simulink model "sim8"  (R2013a)
settings: Solver=ode45  StartTime=0.0  StopTime=10.0  RelTol=1e-3
values from neighbouring files (symbols this model uses):
  a1 = 4    [cwiczenie8.m]    (also in cwiczenie8transmitancja.m)
  A1 = 2    [cwiczenie8.m]    (also in cwiczenie8transmitancja.m; dawid.m)
  A2 = 4    [cwiczenie8.m]    (also in cwiczenie8transmitancja.m; dawid.m)
  a2 = 5    [cwiczenie8.m]    (also in cwiczenie8transmitancja.m)
  czas_skoku = 2    [cwiczenie8.m]    (also in cwiczenie8transmitancja.m; dawid.m)
  du = 0.1*u0max    (= 0.3)    [cwiczenie8.m]    (also in cwiczenie8transmitancja.m; dawid.m)
  h10 = u0/a1    [cwiczenie8.m]    (also in cwiczenie8transmitancja.m; dawid.m = u0*u0 / (Awy*Awy*2*g))
  h20 = u0/a2    [cwiczenie8.m]    (also in cwiczenie8transmitancja.m; dawid.m = u0*u0 / (Awe*Awe*2*g))
  u0 = tabu0(i)    [cwiczenie8.m]    (also in cwiczenie8transmitancja.m; dawid.m)
settings Model: Creator=LAB320-1552  LastModifiedBy=LAB320-1552

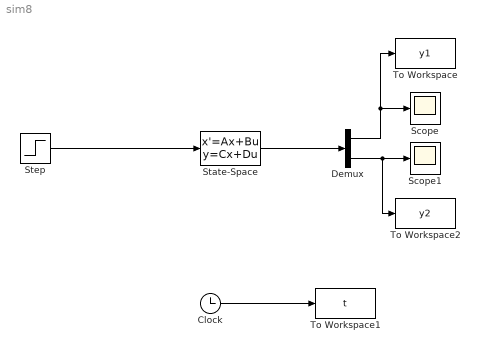
== system sim8 ==
  Clock : Clock
  Demux : Demux  Outputs=2
  Scope : Scope
  Scope1 : Scope
  State-Space : StateSpace  A=[-a1/A1, 0; a1/A2, -a2/A2]  B=[1/A1; 0]  C=[1, 0; 0, 1]  D=[0; 0]  X0=[h10; h20]
  Step : Step  Time=czas_skoku  Before=u0  After=u0+du  SampleTime=0
  To Workspace : ToWorkspace  VariableName=y1  SampleTime=-1
  To Workspace1 : ToWorkspace  VariableName=t  SampleTime=-1
  To Workspace2 : ToWorkspace  VariableName=y2  SampleTime=-1
  wires:
  State-Space/1 -> Demux/1
  Demux/1 -> To Workspace/1, Scope/1
  Step/1 -> State-Space/1
  Clock/1 -> To Workspace1/1
  Demux/2 -> To Workspace2/1, Scope1/1
